simulink model "ADC_FULL"  (Simulink 9.1)
settings: Solver=VariableStepAuto  StartTime=0.0  StopTime=5131  RelTol=1e-3  EnableMultiTasking=on
undefined symbols (not defined in the file or in its folder): magnitude
libraries: F_Line_block x60
settings Model: LogicAnalyzerSignalOrdering=29c98a19-03e6-47c6-b679-a094db8f3ab0,6442f67d-e2a4-42e6-a7b7-5284f6f85cd6  Creator=altari  LastModifiedBy=dongw
settings DataIOCC: LimitDataPoints=on  SaveFormat=Dataset
settings DebuggingCC: UnderspecifiedInitializationDetection=Simplified  MergeDetectMultiDrivingBlocksExec=error  AllowSymbolicDim=off
settings HardwareCC: ProdBitPerPointer=64  ProdBitPerSizeT=64  ProdBitPerPtrDiffT=64  ProdLargestAtomicFloat=Float  ProdIntDivRoundTo=Zero  ProdEndianess=LittleEndian  ProdWordSize=64  ProdHWDeviceType=Intel->x86-64 (Windows64)
settings GRTTargetCC: CombineOutputUpdateFcns=on  GRTInterface=off

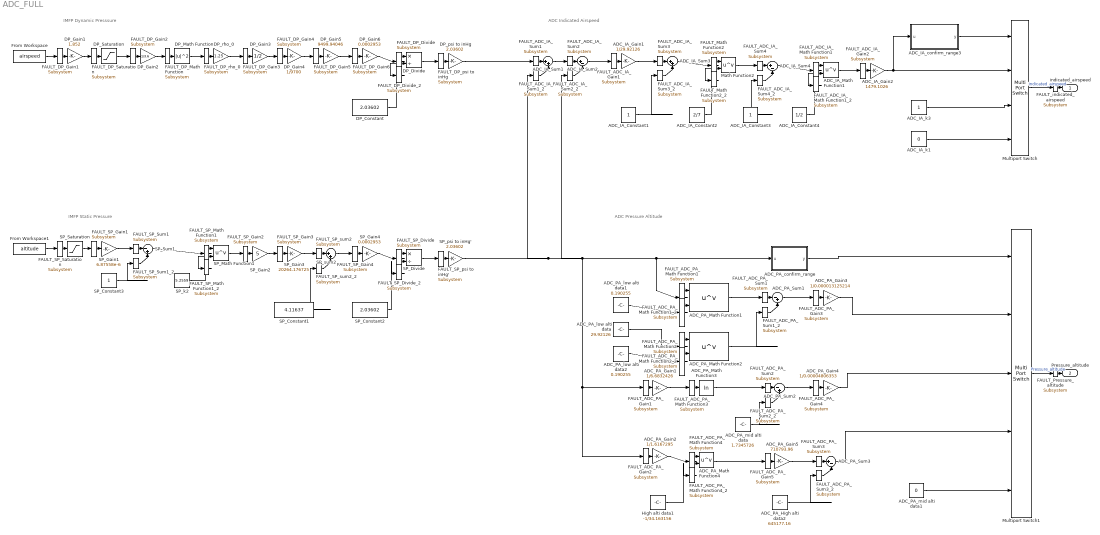
== system ADC_FULL ==
  note: IMFP Dynamic Presssure
  note: IMFP Static Pressure
  note: ADC Indicated Airspeed
  note: ADC Pressure Altitude
  ADC_IA_Constant1 : Constant
  ADC_IA_Constant2 : Constant  Value=2/7
  ADC_IA_Constant3 : Constant
  ADC_IA_Constant4 : Constant  Value=1/2
  ADC_IA_Gain1 : Gain  Gain=1/29.92126
  FAULT_ADC_IA_Gain1 : F_Line_block/Subsystem
  ADC_IA_Gain2 : Gain  Gain=1479.1026
  FAULT_ADC_IA_Gain2 : F_Line_block/Subsystem
  ADC_IA_Math Function1 : Math  Operator=pow  SaturateOnIntegerOverflow=on
  FAULT_ADC_IA_Math Function1 : F_Line_block/Subsystem
  FAULT_ADC_IA_Math Function1_2 : F_Line_block/Subsystem
  ADC_IA_Sum1 : Sum  Inputs=|++
  FAULT_ADC_IA_Sum{1..4} (4 alike) : F_Line_block/Subsystem
  FAULT_ADC_IA_Sum1_2 : F_Line_block/Subsystem
  ADC_IA_Sum2 : Sum  Inputs=|+-
  FAULT_ADC_IA_Sum2_2 : F_Line_block/Subsystem
  ADC_IA_Sum3 : Sum  Inputs=|++
  FAULT_ADC_IA_Sum3_2 : F_Line_block/Subsystem
  ADC_IA_Sum4 : Sum  Inputs=|+-
  FAULT_ADC_IA_Sum4_2 : F_Line_block/Subsystem
  ADC_IA_confirm_range3 : MATLAB Function  TreatAsAtomicUnit=on
  ADC_IA_k1 : Constant  Value=0
  ADC_IA_k3 : Constant
  ADC_PA_Gain1 : Gain  Gain=1/6.6832426
  FAULT_ADC_PA_Gain{1..5} (5 alike) : F_Line_block/Subsystem
  ADC_PA_Gain2 : Gain  Gain=1/1.6167295
  ADC_PA_Gain3 : Gain  Gain=1/0.000013125214
  ADC_PA_Gain4 : Gain  Gain=1/0.00004806353
  ADC_PA_Gain5 : Gain  Gain=710793.96
  ADC_PA_High alti data2 : Constant  Value=645177.16
  ADC_PA_Math Function1 : Math  Operator=pow  SaturateOnIntegerOverflow=on
  FAULT_ADC_PA_Math Function{1..4} (4 alike) : F_Line_block/Subsystem
  FAULT_ADC_PA_Math Function1_2 : F_Line_block/Subsystem
  ADC_PA_Math Function2 : Math  Operator=pow  SaturateOnIntegerOverflow=on
  FAULT_ADC_PA_Math Function2_2 : F_Line_block/Subsystem
  ADC_PA_Math Function3 : Math  Operator=log  SaturateOnIntegerOverflow=on
  ADC_PA_Math Function4 : Math  Operator=pow  SaturateOnIntegerOverflow=on
  FAULT_ADC_PA_Math Function4_2 : F_Line_block/Subsystem
  ADC_PA_Sum1 : Sum  Inputs=|-+
  FAULT_ADC_PA_Sum1 : F_Line_block/Subsystem
  FAULT_ADC_PA_Sum1_2 : F_Line_block/Subsystem
  ADC_PA_Sum2 : Sum  Inputs=|-+
  FAULT_ADC_PA_Sum2 : F_Line_block/Subsystem
  FAULT_ADC_PA_Sum2_2 : F_Line_block/Subsystem
  ADC_PA_Sum3 : Sum  Inputs=|+-
  FAULT_ADC_PA_Sum3 : F_Line_block/Subsystem
  FAULT_ADC_PA_Sum3_2 : F_Line_block/Subsystem
  ADC_PA_confirm_range : MATLAB Function  TreatAsAtomicUnit=on
  ADC_PA_low alti data : Constant  Value=29.92126
  ADC_PA_low alti data1 : Constant  Value=0.190255
  ADC_PA_low alti data2 : Constant  Value=0.190255
  ADC_PA_mid alti data : Constant  Value=1.7345726
  ADC_PA_mid alti data1 : Constant  Value=0
  DP_Constant : Constant  Value=2.03602
  DP_Divide : Product  Inputs=*/
  FAULT_DP_Divide : F_Line_block/Subsystem
  FAULT_DP_Divide_2 : F_Line_block/Subsystem
  DP_Gain1 : Gain  Tag=DP_Gain1  Gain=1.852
  FAULT_DP_Gain{1..6} (6 alike) : F_Line_block/Subsystem
  DP_Gain2 : Gain  Gain=1/3.6
  DP_Gain3 : Gain  Gain=1/2
  DP_Gain4 : Gain  Gain=1/9700
  DP_Gain5 : Gain  Gain=9499.94046
  DP_Gain6 : Gain  Gain=0.0002953
  DP_Math Function : Math  Operator=magnitude^2  SaturateOnIntegerOverflow=on
  FAULT_DP_Math Function : F_Line_block/Subsystem
  DP_Saturation : Saturate  UpperLimit=1000  LowerLimit=0
  FAULT_DP_Saturation : F_Line_block/Subsystem
  DP_psi to inHg : Gain  Gain=2.03602
  FAULT_DP_psi to inHg : F_Line_block/Subsystem
  DP_rho_0 : Gain  Gain=1.25
  FAULT_DP_rho_0 : F_Line_block/Subsystem
  From Workspace : FromWorkspace  VariableName=airspeed  SampleTime=1
  From Workspace1 : FromWorkspace  VariableName=altitude  SampleTime=1
  High alti data1 : Constant  Value=-1/34.163156
  Math Function2 : Math  Operator=pow  SaturateOnIntegerOverflow=on
  FAULT_Math Function2 : F_Line_block/Subsystem
  FAULT_Math Function2_2 : F_Line_block/Subsystem
  Multiport Switch : MultiPortSwitch
  Multiport Switch1 : MultiPortSwitch  Inputs=4
  SP_Constant1 : Constant  Value=4.11637
  SP_Constant2 : Constant  Value=2.03602
  SP_Constant3 : Constant
  SP_Divide : Product  Inputs=*/
  FAULT_SP_Divide : F_Line_block/Subsystem
  FAULT_SP_Divide_2 : F_Line_block/Subsystem
  SP_Gain1 : Gain  Gain=6.87558e-6
  FAULT_SP_Gain{1..4} (4 alike) : F_Line_block/Subsystem
  SP_Gain2 : Gain  Gain=5
  SP_Gain3 : Gain  Gain=20264.176725
  SP_Gain4 : Gain  Gain=0.0002953
  SP_Math Function1 : Math  Operator=pow  SaturateOnIntegerOverflow=on
  FAULT_SP_Math Function1 : F_Line_block/Subsystem
  FAULT_SP_Math Function1_2 : F_Line_block/Subsystem
  SP_Saturation : Saturate  UpperLimit=48000  LowerLimit=0
  FAULT_SP_Saturation : F_Line_block/Subsystem
  SP_Sum1 : Sum  Inputs=|-+
  FAULT_SP_Sum1 : F_Line_block/Subsystem
  FAULT_SP_Sum1_2 : F_Line_block/Subsystem
  SP_k2 : Constant  Value=5.2559
  SP_psi to inHg' : Gain  Gain=2.03602
  FAULT_SP_psi to inHg' : F_Line_block/Subsystem
  SP_sum2 : Sum  Inputs=|++
  FAULT_SP_sum2 : F_Line_block/Subsystem
  FAULT_SP_sum2_2 : F_Line_block/Subsystem
  indicated_airspeed : Outport
  FAULT_indicated_airspeed : F_Line_block/Subsystem
  Pressure_altitude : Outport  Port=2
  FAULT_Pressure_altitude : F_Line_block/Subsystem
  wires:
  Multiport Switch1/1 -> FAULT_Pressure_altitude/1  "Pressure_altitude"
  FAULT_Pressure_altitude/1 -> Pressure_altitude/1
  Multiport Switch/1 -> FAULT_indicated_airspeed/1  "indicated_airspeed"
  FAULT_indicated_airspeed/1 -> indicated_airspeed/1
  DP_Constant/1 -> FAULT_DP_Divide_2/1
  FAULT_DP_Divide_2/1 -> DP_Divide/2
  DP_Gain6/1 -> FAULT_DP_Divide/1
  FAULT_DP_Divide/1 -> DP_Divide/1
  DP_Gain4/1 -> FAULT_DP_Gain5/1
  FAULT_DP_Gain5/1 -> DP_Gain5/1
  DP_Gain5/1 -> FAULT_DP_Gain6/1
  FAULT_DP_Gain6/1 -> DP_Gain6/1
  SP_Constant2/1 -> FAULT_SP_Divide_2/1
  FAULT_SP_Divide_2/1 -> SP_Divide/2
  SP_Gain4/1 -> FAULT_SP_Divide/1
  FAULT_SP_Divide/1 -> SP_Divide/1
  SP_Gain3/1 -> FAULT_SP_sum2/1
  FAULT_SP_sum2/1 -> SP_sum2/1
  SP_Constant1/1 -> FAULT_SP_sum2_2/1
  FAULT_SP_sum2_2/1 -> SP_sum2/2
  SP_sum2/1 -> FAULT_SP_Gain4/1
  FAULT_SP_Gain4/1 -> SP_Gain4/1
  SP_Gain2/1 -> FAULT_SP_Gain3/1
  FAULT_SP_Gain3/1 -> SP_Gain3/1
  From Workspace/1 -> FAULT_DP_Gain1/1
  FAULT_DP_Gain1/1 -> DP_Gain1/1
  SP_Divide/1 -> FAULT_SP_psi to inHg'/1
  FAULT_SP_psi to inHg'/1 -> SP_psi to inHg'/1
  DP_psi to inHg/1 -> FAULT_ADC_IA_Sum1/1
  FAULT_ADC_IA_Sum1/1 -> ADC_IA_Sum1/1
  DP_Divide/1 -> FAULT_DP_psi to inHg/1
  FAULT_DP_psi to inHg/1 -> DP_psi to inHg/1
  ADC_IA_Sum1/1 -> FAULT_ADC_IA_Sum2/1
  FAULT_ADC_IA_Sum2/1 -> ADC_IA_Sum2/1
  ADC_IA_Gain2/1 -> Multiport Switch/2, ADC_IA_confirm_range3/1(u)
  ADC_IA_Math Function1/1 -> FAULT_ADC_IA_Gain2/1
  FAULT_ADC_IA_Gain2/1 -> ADC_IA_Gain2/1
  ADC_IA_Constant4/1 -> FAULT_ADC_IA_Math Function1_2/1
  FAULT_ADC_IA_Math Function1_2/1 -> ADC_IA_Math Function1/2
  ADC_IA_Sum4/1 -> FAULT_ADC_IA_Math Function1/1
  FAULT_ADC_IA_Math Function1/1 -> ADC_IA_Math Function1/1
  Math Function2/1 -> FAULT_ADC_IA_Sum4/1
  FAULT_ADC_IA_Sum4/1 -> ADC_IA_Sum4/1
  ADC_IA_Sum3/1 -> FAULT_Math Function2/1
  FAULT_Math Function2/1 -> Math Function2/1
  ADC_IA_Constant3/1 -> FAULT_ADC_IA_Sum4_2/1
  FAULT_ADC_IA_Sum4_2/1 -> ADC_IA_Sum4/2
  ADC_IA_Sum2/1 -> FAULT_ADC_IA_Gain1/1
  FAULT_ADC_IA_Gain1/1 -> ADC_IA_Gain1/1
  ADC_IA_confirm_range3/1(y) -> Multiport Switch/1
  ADC_IA_k3/1 -> Multiport Switch/3
  ADC_IA_Gain1/1 -> FAULT_ADC_IA_Sum3/1
  FAULT_ADC_IA_Sum3/1 -> ADC_IA_Sum3/1
  ADC_IA_Constant2/1 -> FAULT_Math Function2_2/1
  FAULT_Math Function2_2/1 -> Math Function2/2
  ADC_IA_k1/1 -> Multiport Switch/4
  DP_Gain2/1 -> FAULT_DP_Math Function/1
  FAULT_DP_Math Function/1 -> DP_Math Function/1
  DP_Math Function/1 -> FAULT_DP_rho_0/1
  FAULT_DP_rho_0/1 -> DP_rho_0/1
  DP_Gain1/1 -> FAULT_DP_Saturation/1
  FAULT_DP_Saturation/1 -> DP_Saturation/1
  DP_rho_0/1 -> FAULT_DP_Gain3/1
  FAULT_DP_Gain3/1 -> DP_Gain3/1
  DP_Gain3/1 -> FAULT_DP_Gain4/1
  FAULT_DP_Gain4/1 -> DP_Gain4/1
  DP_Saturation/1 -> FAULT_DP_Gain2/1
  FAULT_DP_Gain2/1 -> DP_Gain2/1
  SP_k2/1 -> FAULT_SP_Math Function1_2/1
  FAULT_SP_Math Function1_2/1 -> SP_Math Function1/2
  SP_Sum1/1 -> FAULT_SP_Math Function1/1
  FAULT_SP_Math Function1/1 -> SP_Math Function1/1
  SP_Constant3/1 -> FAULT_SP_Sum1_2/1
  FAULT_SP_Sum1_2/1 -> SP_Sum1/2
  SP_Gain1/1 -> FAULT_SP_Sum1/1
  FAULT_SP_Sum1/1 -> SP_Sum1/1
  SP_Saturation/1 -> FAULT_SP_Gain1/1
  FAULT_SP_Gain1/1 -> SP_Gain1/1
  SP_Math Function1/1 -> FAULT_SP_Gain2/1
  FAULT_SP_Gain2/1 -> SP_Gain2/1
  From Workspace1/1 -> FAULT_SP_Saturation/1
  FAULT_SP_Saturation/1 -> SP_Saturation/1
  ADC_PA_mid alti data1/1 -> Multiport Switch1/5
  ADC_PA_Sum3/1 -> Multiport Switch1/4
  ADC_PA_High alti data2/1 -> FAULT_ADC_PA_Sum3_2/1
  FAULT_ADC_PA_Sum3_2/1 -> ADC_PA_Sum3/2
  ADC_PA_Gain5/1 -> FAULT_ADC_PA_Sum3/1
  FAULT_ADC_PA_Sum3/1 -> ADC_PA_Sum3/1
  ADC_PA_Math Function4/1 -> FAULT_ADC_PA_Gain5/1
  FAULT_ADC_PA_Gain5/1 -> ADC_PA_Gain5/1
  High alti data1/1 -> FAULT_ADC_PA_Math Function4_2/1
  FAULT_ADC_PA_Math Function4_2/1 -> ADC_PA_Math Function4/2
  ADC_PA_Gain2/1 -> FAULT_ADC_PA_Math Function4/1
  FAULT_ADC_PA_Math Function4/1 -> ADC_PA_Math Function4/1
  ADC_PA_Gain4/1 -> Multiport Switch1/3
  ADC_PA_Sum2/1 -> FAULT_ADC_PA_Gain4/1
  FAULT_ADC_PA_Gain4/1 -> ADC_PA_Gain4/1
  ADC_PA_mid alti data/1 -> FAULT_ADC_PA_Sum2_2/1
  FAULT_ADC_PA_Sum2_2/1 -> ADC_PA_Sum2/2
  ADC_PA_Math Function3/1 -> FAULT_ADC_PA_Sum2/1
  FAULT_ADC_PA_Sum2/1 -> ADC_PA_Sum2/1
  ADC_PA_Gain1/1 -> FAULT_ADC_PA_Math Function3/1
  FAULT_ADC_PA_Math Function3/1 -> ADC_PA_Math Function3/1
  ADC_PA_Gain3/1 -> Multiport Switch1/2
  ADC_PA_Sum1/1 -> FAULT_ADC_PA_Gain3/1
  FAULT_ADC_PA_Gain3/1 -> ADC_PA_Gain3/1
  ADC_PA_Math Function1/1 -> FAULT_ADC_PA_Sum1/1
  FAULT_ADC_PA_Sum1/1 -> ADC_PA_Sum1/1
  ADC_PA_low alti data1/1 -> FAULT_ADC_PA_Math Function1_2/1
  FAULT_ADC_PA_Math Function1_2/1 -> ADC_PA_Math Function1/2
  ADC_PA_Math Function2/1 -> FAULT_ADC_PA_Sum1_2/1
  FAULT_ADC_PA_Sum1_2/1 -> ADC_PA_Sum1/2
  ADC_PA_low alti data2/1 -> FAULT_ADC_PA_Math Function2_2/1
  FAULT_ADC_PA_Math Function2_2/1 -> ADC_PA_Math Function2/2
  ADC_PA_low alti data/1 -> FAULT_ADC_PA_Math Function2/1
  FAULT_ADC_PA_Math Function2/1 -> ADC_PA_Math Function2/1
  ADC_PA_confirm_range/1(y) -> Multiport Switch1/1
  SP_psi to inHg'/1 -> FAULT_ADC_IA_Sum1_2/1, ADC_PA_confirm_range/1(u), FAULT_ADC_PA_Math Function1/1, FAULT_ADC_PA_Gain1/1, FAULT_ADC_PA_Gain2/1, FAULT_ADC_IA_Sum2_2/1
  FAULT_ADC_IA_Sum1_2/1 -> ADC_IA_Sum1/2
  FAULT_ADC_PA_Math Function1/1 -> ADC_PA_Math Function1/1
  FAULT_ADC_PA_Gain1/1 -> ADC_PA_Gain1/1
  FAULT_ADC_PA_Gain2/1 -> ADC_PA_Gain2/1
  FAULT_ADC_IA_Sum2_2/1 -> ADC_IA_Sum2/2
  ADC_IA_Constant1/1 -> FAULT_ADC_IA_Sum3_2/1
  FAULT_ADC_IA_Sum3_2/1 -> ADC_IA_Sum3/2

== matlab function ADC_IA_confirm_range3 ==
  data: u input double; y output double
function y = confirm_range3(u)
%#codegen

if u>0
    if u<661.493
        y=1;
    else
        y=2;
    end
else
    y=3;
end

== matlab function ADC_PA_confirm_range ==
  data: u input double; y output double
function y = confirm_range(u)
%#codegen

if u>0
    if u<=1.617295
        y=3;
    else
        if u<=6.683246
            y=2;
        else
            y=1;
        end
    end
else
    y=-1;
end
